simulink model "keyless_entry_sim"  (R2024a)
settings: Solver=VariableStepAuto  StartTime=0.0  StopTime=15  RelTol=1e-3
libraries: simulink x2
settings Model: Creator=chiemerieokeke  LastModifiedBy=chiemerieokeke

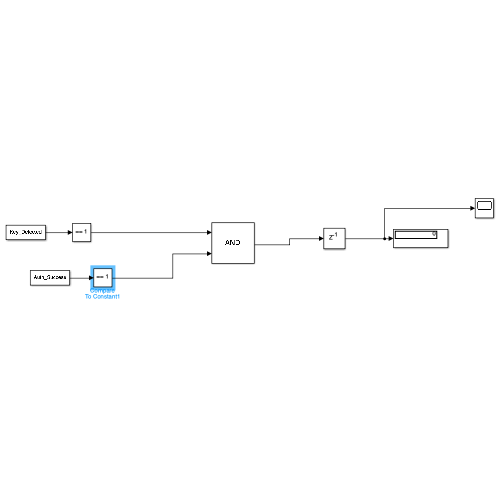
[thumbnail: Simulink's stored preview of the top-level diagram]
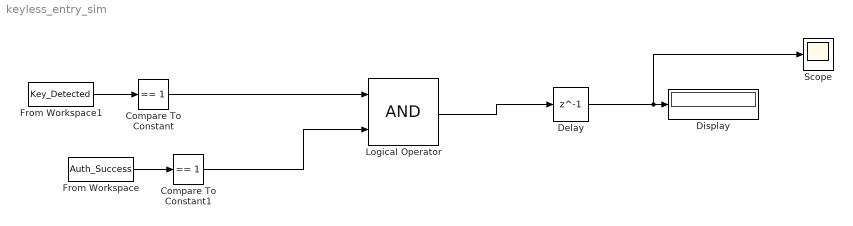
== system keyless_entry_sim ==
  Compare To Constant : simulink/Logic and Bit Operations/Compare To Constant  relop===  const=1  OutDataTypeStr=boolean
  Compare To Constant1 : simulink/Logic and Bit Operations/Compare To Constant  relop===  const=1  OutDataTypeStr=boolean
  Delay : Delay  DelayLength=1  InitialCondition=0
  Display : Display
  From Workspace : FromWorkspace  VariableName=Auth_Success
  From Workspace1 : FromWorkspace  VariableName=Key_Detected
  Logical Operator : Logic  AllPortsSameDT=off  OutDataTypeStr=boolean
  Scope : Scope
  wires:
  From Workspace1/1 -> Compare To Constant/1
  From Workspace/1 -> Compare To Constant1/1
  Compare To Constant/1 -> Logical Operator/1
  Compare To Constant1/1 -> Logical Operator/2
  Delay/1 -> Scope/1, Display/1
  Logical Operator/1 -> Delay/1
